simulink model "B2B_2x15kW_LCO_paralelo_y_serie"  (R2026b)
settings: Solver=ode5  StopTime=inf  EnableMultiTasking=on
StopFcn:
  | Modelo_Disable_B2B
undefined symbols (not defined in the file): ALPHA_DC, COS_RO, dataStateMachine, DiscIntNeverNeededParam, dq2abc, EN_G, getNormalizedOffset, I_MAX_G, INV_SIN_RO, KAW_CCG, KAW_DC, KI_CCG, KI_DC, KI_PLLG, KP_CCG, KP_DC, KP_PLLG, L12, LIMIT_SAG_DETECT, magnitude, MIN_VDC_READY, Ncount, NDELAY_SAG_DETECT, PORC_DC_STEADS, SAMPLES_SAG_DETECT, simDCcontCurrent1, simDCcontCurrent2, SN_G, Transformations_blocks, ts, Ts_al, TS_C, TS_PLL, UDC_min_al, UDC_Ref_al, VDC_REF, WN_G
libraries: simulink x15, TriPhaseDriveControl x13, powerlib_extras x2, model_hardware_PM15F80C_rev x2, TriphaseXenomaiTarget x1
(part 2 of 4)

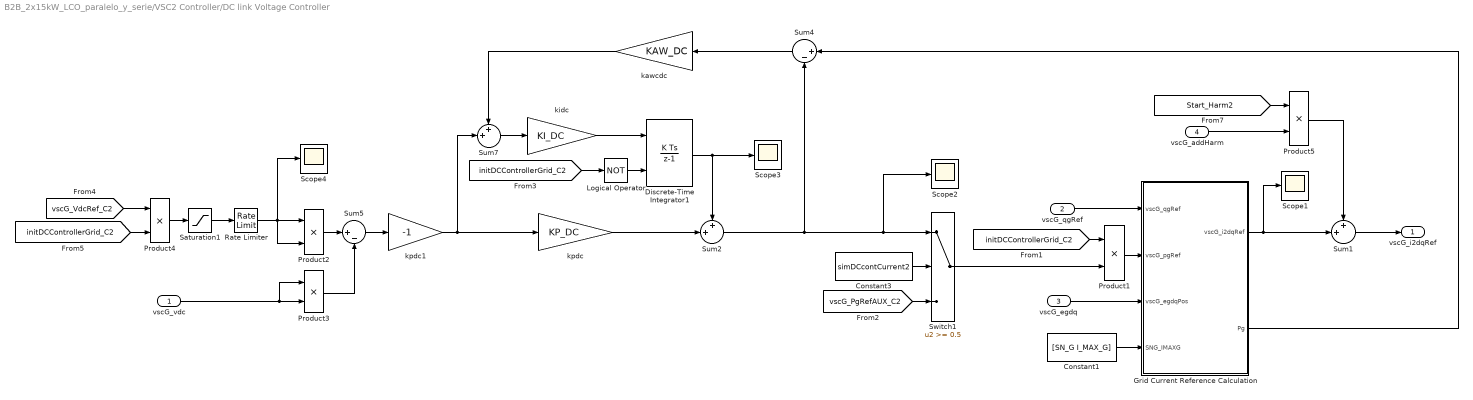
== system B2B_2x15kW_LCO_paralelo_y_serie/VSC2 Controller/DC link Voltage Controller ==
  vscG_vdc : Inport
  vscG_qgRef : Inport  Port=2
  vscG_egdq : Inport  Port=3
  vscG_addHarm : Inport  Port=4
  Constant1 : Constant  Value=[SN_G I_MAX_G]  SampleTime=TS_C
  Constant3 : Constant  Value=simDCcontCurrent2  SampleTime=TS_C
  Discrete-Time Integrator1 : DiscreteIntegrator  ExternalReset=level  SampleTime=-1  UpperSaturationLimit=sqrt(2/3)*750  LowerSaturationLimit=-sqrt(2/3)*750  ICPrevOutput=DiscIntNeverNeededParam  ICPrevScaledInput=DiscIntNeverNeededParam
  Grid Current Reference Calculation : MATLAB Function  TreatAsAtomicUnit=on
  Logical Operator : Logic  Operator=NOT  AllPortsSameDT=off  OutDataTypeStr=boolean
  Product1 : Product  RndMeth=Zero
  Product2 : Product  SaturateOnIntegerOverflow=on  OutDataTypeStr=Inherit: Same as first input
  Product3 : Product  SaturateOnIntegerOverflow=on  OutDataTypeStr=Inherit: Same as first input
  Product4 : Product  SaturateOnIntegerOverflow=on  OutDataTypeStr=Inherit: Same as first input
  Product5 : Product  RndMeth=Zero
  Rate Limiter : RateLimiter  RisingSlewLimit=500/1  FallingSlewLimit=-500/1  SampleTimeMode=inherited  InitialCondition=EN_G*sqrt(2)
  Saturation1 : Saturate  UpperLimit=VDC_REF*1.1  LowerLimit=EN_G*sqrt(2)
  Scope{1..4} (4 alike) : Scope
      Scope1 settings: SampleTime=TS_C  TimeSpan=10  ActiveDisplayYMinimum=-0  ActiveDisplayYMaximum=22  DataLoggingDecimation=5  DataLoggingVariableName=Variables_i2dq2  DataLoggingSaveFormat=Array
      Scope2 settings: SampleTime=TS_C  TimeSpan=5  ActiveDisplayYMinimum=-30000  ActiveDisplayYMaximum=2500  DataLoggingDecimation=5  DataLoggingVariableName=Variables_i2dq4  DataLoggingSaveFormat=Array
      Scope3 settings: SampleTime=TS_C  TimeSpan=5  ActiveDisplayYMinimum=24681.8  ActiveDisplayYMaximum=27279.8  DataLoggingDecimation=5  DataLoggingVariableName=Variables_i2dq5  DataLoggingSaveFormat=Array
      Scope4 settings: SampleTime=TS_C  TimeSpan=5  ActiveDisplayYMinimum=675  ActiveDisplayYMaximum=680  DataLoggingDecimation=5  DataLoggingVariableName=Variables_i2dq6  DataLoggingSaveFormat=Array
  Sum1 : Sum  Inputs=++|  InputSameDT=on  SaturateOnIntegerOverflow=on  OutDataTypeStr=Inherit: Same as first input
  Sum2 : Sum  Inputs=++|  InputSameDT=on  SaturateOnIntegerOverflow=on  OutDataTypeStr=Inherit: Same as first input
  Sum4 : Sum  Inputs=|+-  InputSameDT=on  SaturateOnIntegerOverflow=on  OutDataTypeStr=Inherit: Same as first input
  Sum5 : Sum  Inputs=|+-  InputSameDT=on  SaturateOnIntegerOverflow=on  OutDataTypeStr=Inherit: Same as first input
  Sum7 : Sum  Inputs=++|  InputSameDT=on  SaturateOnIntegerOverflow=on  OutDataTypeStr=Inherit: Same as first input
  Switch1 : Switch  Threshold=0.5  SaturateOnIntegerOverflow=off  InputSameDT=off
  kawcdc : Gain  Gain=KAW_DC  SaturateOnIntegerOverflow=on  OutDataTypeStr=Inherit: Same as input  ParamDataTypeStr=Inherit: Same as input
  kidc : Gain  Gain=KI_DC  SaturateOnIntegerOverflow=on  OutDataTypeStr=Inherit: Same as input  ParamDataTypeStr=Inherit: Same as input
  kpdc : Gain  Gain=KP_DC  SaturateOnIntegerOverflow=on  OutDataTypeStr=Inherit: Same as input  ParamDataTypeStr=Inherit: Same as input
  kpdc1 : Gain  Gain=-1  SaturateOnIntegerOverflow=on  OutDataTypeStr=Inherit: Same as input  ParamDataTypeStr=Inherit: Same as input
  vscG_i2dqRef : Outport
  wires:
  kidc/1 -> Discrete-Time Integrator1/1
  Grid Current Reference Calculation/1(vscG_i2dqRef) -> Sum1/2, Scope1/1
  vscG_egdq/1 -> Grid Current Reference Calculation/3(vscG_egdqPos)
  Constant1/1 -> Grid Current Reference Calculation/4(SNG_IMAXG)
  Logical Operator/1 -> Discrete-Time Integrator1/2
  [initDCControllerGrid_C2] -> Logical Operator/1
  [initDCControllerGrid_C2] -> Product1/1
  Product1/1 -> Grid Current Reference Calculation/2(vscG_pgRef)
  Constant3/1 -> Switch1/2
  [vscG_PgRefAUX_C2] -> Switch1/3
  Sum5/1 -> kpdc1/1
  Product3/1 -> Sum5/2
  Product2/1 -> Sum5/1
  vscG_vdc/1 -> Product3/1, Product3/2
  kpdc/1 -> Sum2/2
  Discrete-Time Integrator1/1 -> Scope3/1, Sum2/1
  Sum7/1 -> kidc/1
  Sum2/1 -> Sum4/2, Scope2/1, Switch1/1
  Sum4/1 -> kawcdc/1
  kawcdc/1 -> Sum7/1
  Grid Current Reference Calculation/2(Pg) -> Sum4/1
  vscG_qgRef/1 -> Grid Current Reference Calculation/1(vscG_qgRef)
  Switch1/1 -> Product1/2
  kpdc1/1 -> Sum7/2, kpdc/1
  Rate Limiter/1 -> Scope4/1, Product2/2, Product2/1
  [vscG_VdcRef_C2] -> Product4/1
  [initDCControllerGrid_C2] -> Product4/2
  Product4/1 -> Saturation1/1
  Saturation1/1 -> Rate Limiter/1
  vscG_addHarm/1 -> Product5/2
  Product5/1 -> Sum1/1
  [Start_Harm2] -> Product5/1
  Sum1/1 -> vscG_i2dqRef/1

== system B2B_2x15kW_LCO_paralelo_y_serie/VSC2 Controller/Grid Side Measurements ==
  vscG_i1abc : Inport
  vscG_i2abc : Inport  Port=2
  vscG_egabc : Inport  Port=3
  vscG_vdc_ : Inport  Port=4
  DSOGI QSG PLL : Subsystem
  abc to dq eg : Subsystem
  abc to dq i1 : Subsystem
  abc to dq i2 : Subsystem
  udc measurement : Subsystem
  vscG_i1dq : Outport
  vscG_i2dq : Outport  Port=2
  vscG_egdqPos : Outport  Port=3  SampleTime=TS_C
  vscG_thetaPLL : Outport  Port=4  SampleTime=TS_C
  vscG_vdc : Outport  Port=5
  vscG_egdq : Outport  Port=6
  vscG_omegaPLL : Outport  Port=7  SampleTime=TS_C
  wires:
  vscG_i1abc/1 -> abc to dq i1/1(vscG_i1abc)
  vscG_egabc/1 -> abc to dq eg/1(vscG_egabc), DSOGI QSG PLL/1(vscG_egabc)
  vscG_i2abc/1 -> abc to dq i2/1(vscG_i2abc)
  DSOGI QSG PLL/2(vscG_egdqPos) -> vscG_egdqPos/1
  vscG_vdc_/1 -> udc measurement/1(vscG_vdc_)
  udc measurement/1(vscG_vdc) -> vscG_vdc/1
  abc to dq eg/1(vscG_egdq) -> vscG_egdq/1
  DSOGI QSG PLL/3(vscG_omegaPLL) -> vscG_omegaPLL/1
  abc to dq i2/1(vscG_i2dq) -> vscG_i2dq/1
  abc to dq i1/1(vscG_i1dq) -> vscG_i1dq/1
  DSOGI QSG PLL/1(vscG_thetaPLL) -> vscG_thetaPLL/1, abc to dq eg/2(vscG_theta), abc to dq i2/2(vscG_theta), abc to dq i1/2(vscG_theta)

== system B2B_2x15kW_LCO_paralelo_y_serie/VSC2 Controller/Normalizacion ==
  vscG_ugabcActD : Inport
  vscG_vdc : Inport  Port=2
  Demux : Demux  Outputs=3
  Fcn : Fcn  Expr=2*u[1]/(u[2]+eps)
  Fcn1 : Fcn  Expr=2*u[1]/(u[2]+eps)
  Fcn2 : Fcn  Expr=2*u[1]/(u[2]+eps)
  Filter vdc : Subsystem
  Gain1 : Gain  Gain=1/2  SaturateOnIntegerOverflow=on  OutDataTypeStr=Inherit: Same as input  ParamDataTypeStr=Inherit: Same as input
  Manual Switch : ManualSwitch  CurrentSetting=0
  MinMax : MinMax  Function=max  Inputs=3  InputSameDT=on  SaturateOnIntegerOverflow=on
  MinMax2 : MinMax  Inputs=3  InputSameDT=on  SaturateOnIntegerOverflow=on
  Mux1 : Mux  Inputs=2
  Mux2 : Mux  Inputs=2
  Mux3 : Mux  Inputs=2
  Mux4 : Mux  Inputs=3
  Mux5 : Mux  Inputs=3
  Sum2 : Sum  InputSameDT=on  SaturateOnIntegerOverflow=on  OutDataTypeStr=Inherit: Same as first input
  Sum3 : Sum  Inputs=+-  InputSameDT=on  SaturateOnIntegerOverflow=on  OutDataTypeStr=Inherit: Same as first input
  Sum4 : Sum  Inputs=+-  InputSameDT=on  SaturateOnIntegerOverflow=on  OutDataTypeStr=Inherit: Same as first input
  Sum5 : Sum  Inputs=+-  InputSameDT=on  SaturateOnIntegerOverflow=on  OutDataTypeStr=Inherit: Same as first input
  vscG_dabc : Outport
  wires:
  vscG_vdc/1 -> Filter vdc/1(vscG_vdc)
  Sum3/1 -> Mux4/1  "vscG_pwmA"
  Sum4/1 -> Mux4/2  "vscG_pwmB"
  Sum5/1 -> Mux4/3  "vscG_pwmC"
  MinMax/1 -> Sum2/1
  MinMax2/1 -> Sum2/2
  Sum2/1 -> Gain1/1
  Fcn/1 -> Mux5/1, Sum3/1, MinMax2/1, MinMax/1
  Fcn2/1 -> MinMax/3, MinMax2/3, Sum5/1, Mux5/3
  Fcn1/1 -> Mux5/2, MinMax/2, MinMax2/2, Sum4/1
  Mux1/1 -> Fcn/1
  Mux2/1 -> Fcn1/1
  Mux3/1 -> Fcn2/1
  Demux/2 -> Mux2/1
  Demux/3 -> Mux3/1
  Demux/1 -> Mux1/1
  Gain1/1 -> Sum3/2, Sum4/2, Sum5/2
  Filter vdc/1(Out) -> Mux3/2, Mux1/2, Mux2/2
  vscG_ugabcActD/1 -> Demux/1
  Mux4/1 -> Manual Switch/2
  Mux5/1 -> Manual Switch/1
  Manual Switch/1 -> vscG_dabc/1

== system B2B_2x15kW_LCO_paralelo_y_serie/VSC2 Controller/State Machine ==
  Constant2 : Constant  Value=dataStateMachine  SampleTime=TS_C
  Constant6 : Constant  SampleTime=TS_C
  Constant8 : Constant  Value=0  SampleTime=TS_C
  Demux : Demux  Outputs=8
  Logic detection : Subsystem
  Mux : Mux  Inputs=6
  Scope2 : Scope
      settings: ActiveDisplayYMinimum=0  ActiveDisplayYMaximum=2100  DataLoggingVariableName=ScopeData12
  Scope3 : Scope
      settings: ActiveDisplayYMinimum=1.9  ActiveDisplayYMaximum=2.1  DataLoggingVariableName=ScopeData14
  State Machine : MATLAB Function  TreatAsAtomicUnit=on
  Unit Delay5 : UnitDelay  InitialCondition=zeros(1,Ncount)  SampleTime=TS_C
  Unit Delay7 : UnitDelay  InitialCondition=1  SampleTime=TS_C
  tag scope: CONNECT_GRID_CONTACT_C2=global, CONNECT_PRELOAD_CONTACT_C2=global, PWMOnGrid_C2=global, initCurrentControllerG_C2=global, initDCControllerGrid_C2=global, initPLLGrid_C2=global, initReactiveVoltageController_C2=global, selReactiveVoltageController_C2=global
  wires:
  State Machine/3(nowCounters) -> Unit Delay5/1, Scope2/1
  Mux/1 -> State Machine/2(inputs)
  Constant2/1 -> State Machine/1(data)
  Unit Delay5/1 -> State Machine/4(prevCounters)
  State Machine/2(nowState) -> Unit Delay7/1, Scope3/1
  Unit Delay7/1 -> State Machine/3(prevState)
  [MEAS_vscG_vdc_C2] -> Logic detection/1(vscG_vdc)
  State Machine/1(outputs) -> Demux/1
  [MEAS_vscG_egabc_C2] -> Logic detection/2(vscG_egabc)
  Demux/1 -> [PWMOnGrid_C2]
  Demux/2 -> [CONNECT_GRID_CONTACT_C2]
  Demux/3 -> [CONNECT_PRELOAD_CONTACT_C2]
  Demux/8 -> [initDCControllerGrid_C2]
  Demux/7 -> [initCurrentControllerG_C2]
  Demux/6 -> [initReactiveVoltageController_C2]
  Demux/5 -> [initPLLGrid_C2]
  Demux/4 -> [selReactiveVoltageController_C2]
  Constant6/1 -> Mux/1  "PRECHARGE"
  [INPUT_CONNECT_INT_C2] -> Mux/2  "CONNECT"
  Constant8/1 -> Mux/3
  Logic detection/1(VDC_READY) -> Mux/4
  Logic detection/2(VDC_STEATS) -> Mux/5
  Logic detection/3(FLAG_SAG) -> Mux/6

== system B2B_2x15kW_LCO_paralelo_y_serie/VSC2 Controller/dq to abc ==
  vscG_ugdqRef : Inport
  vscG_egdqPos : Inport  Port=2
  vscG_theta : Inport  Port=3
  Constant : Constant  Value=[WN_G L12 I_MAX_G]  SampleTime=TS_C
  Constant1 : Constant  Value=WN_G  SampleTime=TS_C
  Mux : Mux  Inputs=2
  Scope3 : Scope
      settings: SampleTime=TS_C  TimeSpan=5  ActiveDisplayYMinimum=24681.8  ActiveDisplayYMaximum=27279.8  DataLoggingDecimation=5  DataLoggingVariableName=Variables_i2dq7  DataLoggingSaveFormat=Array
  Sum : Sum  Inputs=|++
  dq to abc : Subsystem  AncestorBlock=Transformations_blocks/dq2abc
  th advance : Gain  Gain=TS_C*5/2
  udq Limitation : MATLAB Function  TreatAsAtomicUnit=on
  vscG_ugabcSat : Outport
  vscG_ugdqSat : Outport  Port=2
  wires:
  dq to abc/1(vscG_ugabcSat) -> vscG_ugabcSat/1
  Sum/1 -> dq to abc/2(vsc_thetaAdvanced)
  vscG_theta/1 -> Sum/1
  th advance/1 -> Sum/2
  Constant1/1 -> th advance/1
  Constant/1 -> udq Limitation/3(WNG_L12_IMAXG)
  vscG_egdqPos/1 -> udq Limitation/2(vscG_egdqPos)
  udq Limitation/1(vscG_ugdqSat) -> Mux/2, vscG_ugdqSat/1, dq to abc/1(vscG_ugdqSat)
  vscG_ugdqRef/1 -> Mux/1, udq Limitation/1(vscG_ugdqRef)
  Mux/1 -> Scope3/1

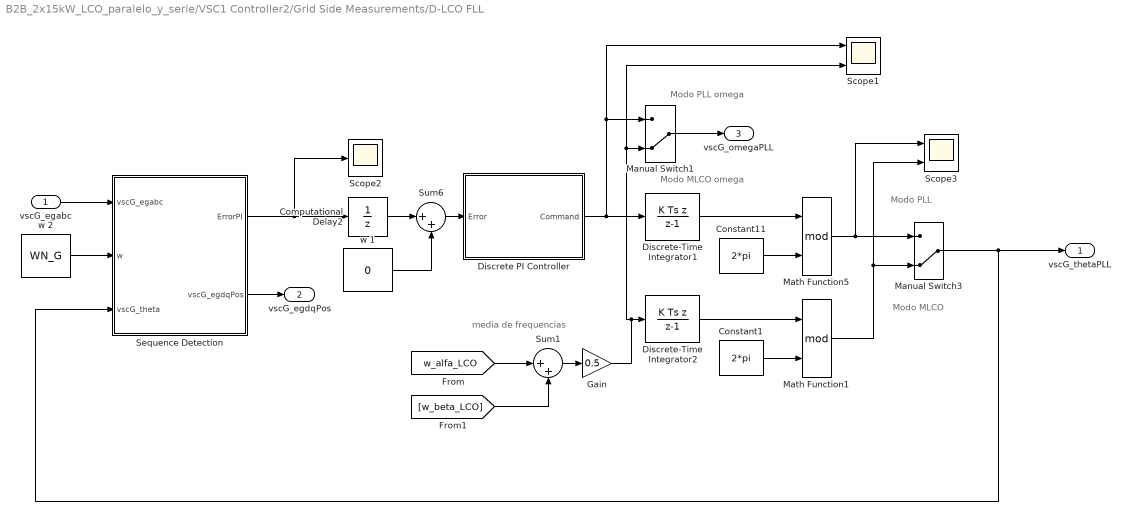
== system B2B_2x15kW_LCO_paralelo_y_serie/VSC1 Controller2/Grid Side Measurements/D-LCO FLL ==
  note: media de frequencias
  note: Modo MLCO omega
  note: Modo PLL
  note: Modo MLCO
  note: Modo PLL omega
  vscG_egabc : Inport  SampleTime=TS_PLL
  Computational Delay2 : UnitDelay  SampleTime=-1
  Constant1 : Constant  Value=2*pi  SampleTime=TS_PLL
  Constant11 : Constant  Value=2*pi  SampleTime=TS_PLL
  Discrete PI Controller : Subsystem
  Discrete-Time Integrator1 : DiscreteIntegrator  IntegratorMethod=Integration: Backward Euler  gainval=1  SampleTime=-1  ICPrevOutput=DiscIntNeverNeededParam  ICPrevScaledInput=DiscIntNeverNeededParam
  Discrete-Time Integrator2 : DiscreteIntegrator  IntegratorMethod=Integration: Backward Euler  gainval=1  SampleTime=-1  ICPrevOutput=DiscIntNeverNeededParam  ICPrevScaledInput=DiscIntNeverNeededParam
  Gain : Gain  Gain=0.5
  Manual Switch1 : ManualSwitch  CurrentSetting=0
  Manual Switch3 : ManualSwitch  CurrentSetting=0
  Math Function1 : Math  Operator=mod  SignedPower=on
  Math Function5 : Math  Operator=mod  SignedPower=on
  Scope1 : Scope  NumInputPorts=2
      settings: SampleTime=TS_C  TimeSpan=0.04  ActiveDisplayYMinimum=426200  ActiveDisplayYMaximum=426800  DataLoggingDecimation=5  DataLoggingVariableName=Variables_i2dq1  DataLoggingSaveFormat=Array
  Scope2 : Scope
      settings: SampleTime=TS_C  TimeSpan=1.978350945590096  ActiveDisplayYMinimum=-0.004  ActiveDisplayYMaximum=0.004  DataLoggingDecimation=5  DataLoggingVariableName=Variables_i2dq3  DataLoggingSaveFormat=Array
  Scope3 : Scope  NumInputPorts=2
      settings: SampleTime=TS_C  TimeSpan=0.08  ActiveDisplayYMinimum=0  ActiveDisplayYMaximum=7  DataLoggingDecimation=5  DataLoggingVariableName=Variables_i2dq  DataLoggingSaveFormat=Array
  Sequence Detection : Subsystem
  Sum1 : Sum  Inputs=|++  InputSameDT=on  SaturateOnIntegerOverflow=on  OutDataTypeStr=Inherit: Same as first input
  Sum6 : Sum  Inputs=|++  InputSameDT=on  SaturateOnIntegerOverflow=on  OutDataTypeStr=Inherit: Same as first input
  w 1 : Constant  Value=0  SampleTime=TS_PLL
  w 2 : Constant  Value=WN_G  SampleTime=TS_PLL
  vscG_thetaPLL : Outport
  vscG_egdqPos : Outport  Port=2
  vscG_omegaPLL : Outport  Port=3
  wires:
  Discrete-Time Integrator2/1 -> Math Function1/1
  Manual Switch1/1 -> vscG_omegaPLL/1
  Math Function1/1 -> Manual Switch3/2, Scope3/2
  Constant1/1 -> Math Function1/2
  Sum1/1 -> Gain/1
  Math Function5/1 -> Manual Switch3/1, Scope3/1
  Constant11/1 -> Math Function5/2
  Discrete-Time Integrator1/1 -> Math Function5/1
  Sum6/1 -> Discrete PI Controller/1(Error)
  Sequence Detection/1(ErrorPI) -> Scope2/1, Computational Delay2/1
  Discrete PI Controller/1(Command) -> Discrete-Time Integrator1/1, Manual Switch1/1, Scope1/1
  Sequence Detection/2(vscG_egdqPos) -> vscG_egdqPos/1
  Manual Switch3/1 -> vscG_thetaPLL/1, Sequence Detection/3(vscG_theta)
  Computational Delay2/1 -> Sum6/1
  vscG_egabc/1 -> Sequence Detection/1(vscG_egabc)
  w 2/1 -> Sequence Detection/2(w)
  w 1/1 -> Sum6/2
  [w_alfa_LCO] -> Sum1/1
  [w_beta_LCO] -> Sum1/2
  Gain/1 -> Manual Switch1/2, Scope1/2, Discrete-Time Integrator2/1

== system B2B_2x15kW_LCO_paralelo_y_serie/VSC1 Controller2/Grid Side Measurements/abc to dq eg ==
  vscG_egabc : Inport  SampleTime=TS_C
  vscG_theta : Inport  Port=2  SampleTime=TS_C
  Fcn3 : Fcn  Expr=u[1]*cos(u[3])+u[2]*sin(u[3])
  Fcn4 : Fcn  Expr=-u[1]*sin(u[3])+u[2]*cos(u[3])
  Fcn5 : Fcn  Expr=2/3*(u[1]-1/2*u[2]-1/2*u[3])
  Fcn6 : Fcn  Expr=2/3*(sqrt(3)/2*u[2]-sqrt(3)/2*u[3])
  Mux2 : Mux  Inputs=3
  Mux6 : Mux  Inputs=2
  vscG_egdq : Outport
  wires:
  Fcn5/1 -> Mux2/1
  Fcn6/1 -> Mux2/2
  Fcn4/1 -> Mux6/2
  Fcn3/1 -> Mux6/1
  Mux6/1 -> vscG_egdq/1
  Mux2/1 -> Fcn4/1, Fcn3/1
  vscG_egabc/1 -> Fcn6/1, Fcn5/1
  vscG_theta/1 -> Mux2/3

== system B2B_2x15kW_LCO_paralelo_y_serie/VSC1 Controller2/Grid Side Measurements/abc to dq i1 ==
  vscG_i1abc : Inport
  vscG_theta : Inport  Port=2  SampleTime=TS_C
  Fcn3 : Fcn  Expr=u[1]*cos(u[3])+u[2]*sin(u[3])
  Fcn4 : Fcn  Expr=-u[1]*sin(u[3])+u[2]*cos(u[3])
  Fcn5 : Fcn  Expr=2/3*(u[1]-1/2*u[2]-1/2*u[3])
  Fcn6 : Fcn  Expr=2/3*(sqrt(3)/2*u[2]-sqrt(3)/2*u[3])
  Mux2 : Mux  Inputs=3
  Mux6 : Mux  Inputs=2
  vscG_i1dq : Outport
  wires:
  vscG_i1abc/1 -> Fcn6/1, Fcn5/1
  Mux2/1 -> Fcn3/1, Fcn4/1
  Mux6/1 -> vscG_i1dq/1
  Fcn3/1 -> Mux6/1
  Fcn4/1 -> Mux6/2
  Fcn6/1 -> Mux2/2
  Fcn5/1 -> Mux2/1
  vscG_theta/1 -> Mux2/3

== system B2B_2x15kW_LCO_paralelo_y_serie/VSC1 Controller2/Grid Side Measurements/abc to dq i2 ==
  vscG_i2abc : Inport
  vscG_theta : Inport  Port=2  SampleTime=TS_C
  Fcn5 : Fcn  Expr=2/3*(u[1]-1/2*u[2]-1/2*u[3])
  Fcn6 : Fcn  Expr=2/3*(sqrt(3)/2*u[2]-sqrt(3)/2*u[3])
  Mux2 : Mux  Inputs=3
  Mux6 : Mux  Inputs=2
  d : Fcn  Expr=u[1]*cos(u[3])+u[2]*sin(u[3])
  q : Fcn  Expr=-u[1]*sin(u[3])+u[2]*cos(u[3])
  vscG_i2dq : Outport
  wires:
  vscG_i2abc/1 -> Fcn5/1, Fcn6/1
  Mux2/1 -> d/1, q/1
  Mux6/1 -> vscG_i2dq/1
  d/1 -> Mux6/1
  q/1 -> Mux6/2
  Fcn6/1 -> Mux2/2
  Fcn5/1 -> Mux2/1
  vscG_theta/1 -> Mux2/3

== system B2B_2x15kW_LCO_paralelo_y_serie/VSC1 Controller2/Grid Side Measurements/udc measurement ==
  note: For simulation only,
      | to avoid algebraic loop
  vscG_vdc_ : Inport
  Unit Delay1 : UnitDelay  InitialCondition=VDC_REF  SampleTime=-1
  vscG_vdc : Outport
  tag scope: MEAS_vscG_vdc_C1=global
  wires:
  Unit Delay1/1 -> [MEAS_vscG_vdc_C1], vscG_vdc/1
  vscG_vdc_/1 -> Unit Delay1/1

== system B2B_2x15kW_LCO_paralelo_y_serie/VSC1 Controller2/Normalizacion/Filter vdc ==
  vscG_vdc : Inport
  Gain2 : Gain  Gain=(1-ALPHA_DC)^2
  Gain3 : Gain  Gain=ALPHA_DC
  Gain5 : Gain  Gain=ALPHA_DC
  Sum1 : Sum
  Sum2 : Sum
  Unit Delay2 : UnitDelay  SampleTime=-1
  Unit Delay3 : UnitDelay  SampleTime=-1
  Out : Outport  PortDimensions=1
  wires:
  Gain3/1 -> Sum1/1
  Unit Delay2/1 -> Gain3/1
  Sum1/1 -> Unit Delay2/1, Sum2/2
  Gain2/1 -> Sum1/2
  vscG_vdc/1 -> Gain2/1
  Sum2/1 -> Unit Delay3/1, Out/1
  Unit Delay3/1 -> Gain5/1
  Gain5/1 -> Sum2/1

== system B2B_2x15kW_LCO_paralelo_y_serie/VSC1 Controller2/State Machine/Logic detection ==
  vscG_vdc : Inport  SampleTime=TS_C
  vscG_egabc : Inport  Port=2  SampleTime=TS_C
  Logic Conditions  VDC : Subsystem
  Sag Detection : Subsystem
  VDC_READY : Outport  SampleTime=TS_C
  VDC_STEATS : Outport  Port=2  SampleTime=TS_C
  FLAG_SAG : Outport  Port=3  SampleTime=TS_C
  wires:
  vscG_vdc/1 -> Logic Conditions  VDC/1(vscG_vdc)
  Logic Conditions  VDC/1(VDC_READY) -> VDC_READY/1
  Sag Detection/1(FLAG_SAG) -> FLAG_SAG/1
  vscG_egabc/1 -> Sag Detection/1(vscG_egabc)
  Logic Conditions  VDC/2(VDC_STEADS) -> VDC_STEATS/1

== system B2B_2x15kW_LCO_paralelo_y_serie/VSC1 Controller2/dq to abc/dq to abc ==
  vscG_ugdqSat : Inport
  vsc_thetaAdvanced : Inport  Port=2
  Mux : Mux  Inputs=2
  Mux1 : Mux  Inputs=2
  Mux2 : Mux  Inputs=3
  a : Fcn  Expr=u(1)
  alpha : Fcn  Expr=cos(u(3))*u(1)-sin(u(3))*u(2)
  b : Fcn  Expr=-0.5*u(1)+sin(2*pi/3)*u(2)
  beta : Fcn  Expr=cos(u(3))*u(2)+sin(u(3))*u(1)
  c : Fcn  Expr=-0.5*u(1)-sin(2*pi/3)*u(2)
  vscG_ugabcSat : Outport
  wires:
  Mux2/1 -> vscG_ugabcSat/1
  Mux1/1 -> c/1, b/1, a/1
  vscG_ugdqSat/1 -> Mux/1
  Mux/1 -> alpha/1, beta/1
  alpha/1 -> Mux1/1
  beta/1 -> Mux1/2
  c/1 -> Mux2/3
  b/1 -> Mux2/2
  a/1 -> Mux2/1
  vsc_thetaAdvanced/1 -> Mux/2

== system B2B_2x15kW_LCO_paralelo_y_serie/VSC2 Controller/Grid Side Measurements/DSOGI QSG PLL ==
  vscG_egabc : Inport  SampleTime=TS_PLL
  Computational Delay2 : UnitDelay  SampleTime=-1
  Constant11 : Constant  Value=2*pi  SampleTime=TS_PLL
  Discrete PI Controller : Subsystem
  Discrete-Time Integrator1 : DiscreteIntegrator  IntegratorMethod=Integration: Backward Euler  gainval=1  SampleTime=-1  ICPrevOutput=DiscIntNeverNeededParam  ICPrevScaledInput=DiscIntNeverNeededParam
  Math Function5 : Math  Operator=mod  SignedPower=on
  Scope1 : Scope
      settings: SampleTime=TS_C  TimeSpan=0.04  ActiveDisplayYMinimum=292.5  ActiveDisplayYMaximum=330  DataLoggingDecimation=5  DataLoggingVariableName=Variables_i2dq1  DataLoggingSaveFormat=Array
  Scope2 : Scope
      settings: SampleTime=TS_C  TimeSpan=1.978350945590096  ActiveDisplayYMinimum=-0.05  ActiveDisplayYMaximum=0.045  DataLoggingDecimation=5  DataLoggingVariableName=Variables_i2dq3  DataLoggingSaveFormat=Array
  Sequence Detection : Subsystem
  Sum6 : Sum  Inputs=|++  InputSameDT=on  SaturateOnIntegerOverflow=on  OutDataTypeStr=Inherit: Same as first input
  w 1 : Constant  Value=0  SampleTime=TS_PLL
  w 2 : Constant  Value=WN_G  SampleTime=TS_PLL
  vscG_thetaPLL : Outport
  vscG_egdqPos : Outport  Port=2
  vscG_omegaPLL : Outport  Port=3
  wires:
  Constant11/1 -> Math Function5/2
  Discrete-Time Integrator1/1 -> Math Function5/1
  Sum6/1 -> Discrete PI Controller/1(Error)
  Sequence Detection/1(ErrorPI) -> Scope2/1, Computational Delay2/1
  Discrete PI Controller/1(Command) -> Discrete-Time Integrator1/1, Scope1/1, vscG_omegaPLL/1
  Sequence Detection/2(vscG_egdqPos) -> vscG_egdqPos/1
  Math Function5/1 -> vscG_thetaPLL/1, Sequence Detection/3(vscG_theta)
  Computational Delay2/1 -> Sum6/1
  vscG_egabc/1 -> Sequence Detection/1(vscG_egabc)
  w 2/1 -> Sequence Detection/2(w)
  w 1/1 -> Sum6/2

== system B2B_2x15kW_LCO_paralelo_y_serie/VSC2 Controller/Grid Side Measurements/abc to dq eg ==
  vscG_egabc : Inport  SampleTime=TS_C
  vscG_theta : Inport  Port=2  SampleTime=TS_C
  Fcn3 : Fcn  Expr=u[1]*cos(u[3])+u[2]*sin(u[3])
  Fcn4 : Fcn  Expr=-u[1]*sin(u[3])+u[2]*cos(u[3])
  Fcn5 : Fcn  Expr=2/3*(u[1]-1/2*u[2]-1/2*u[3])
  Fcn6 : Fcn  Expr=2/3*(sqrt(3)/2*u[2]-sqrt(3)/2*u[3])
  Mux2 : Mux  Inputs=3
  Mux6 : Mux  Inputs=2
  vscG_egdq : Outport
  wires:
  Fcn5/1 -> Mux2/1
  Fcn6/1 -> Mux2/2
  Fcn4/1 -> Mux6/2
  Fcn3/1 -> Mux6/1
  Mux6/1 -> vscG_egdq/1
  Mux2/1 -> Fcn4/1, Fcn3/1
  vscG_egabc/1 -> Fcn6/1, Fcn5/1
  vscG_theta/1 -> Mux2/3

== system B2B_2x15kW_LCO_paralelo_y_serie/VSC2 Controller/Grid Side Measurements/abc to dq i1 ==
  vscG_i1abc : Inport
  vscG_theta : Inport  Port=2  SampleTime=TS_C
  Fcn3 : Fcn  Expr=u[1]*cos(u[3])+u[2]*sin(u[3])
  Fcn4 : Fcn  Expr=-u[1]*sin(u[3])+u[2]*cos(u[3])
  Fcn5 : Fcn  Expr=2/3*(u[1]-1/2*u[2]-1/2*u[3])
  Fcn6 : Fcn  Expr=2/3*(sqrt(3)/2*u[2]-sqrt(3)/2*u[3])
  Mux2 : Mux  Inputs=3
  Mux6 : Mux  Inputs=2
  vscG_i1dq : Outport
  wires:
  vscG_i1abc/1 -> Fcn6/1, Fcn5/1
  Mux2/1 -> Fcn3/1, Fcn4/1
  Mux6/1 -> vscG_i1dq/1
  Fcn3/1 -> Mux6/1
  Fcn4/1 -> Mux6/2
  Fcn6/1 -> Mux2/2
  Fcn5/1 -> Mux2/1
  vscG_theta/1 -> Mux2/3

== system B2B_2x15kW_LCO_paralelo_y_serie/VSC2 Controller/Grid Side Measurements/abc to dq i2 ==
  vscG_i2abc : Inport
  vscG_theta : Inport  Port=2  SampleTime=TS_C
  Fcn5 : Fcn  Expr=2/3*(u[1]-1/2*u[2]-1/2*u[3])
  Fcn6 : Fcn  Expr=2/3*(sqrt(3)/2*u[2]-sqrt(3)/2*u[3])
  Mux2 : Mux  Inputs=3
  Mux6 : Mux  Inputs=2
  d : Fcn  Expr=u[1]*cos(u[3])+u[2]*sin(u[3])
  q : Fcn  Expr=-u[1]*sin(u[3])+u[2]*cos(u[3])
  vscG_i2dq : Outport
  wires:
  vscG_i2abc/1 -> Fcn5/1, Fcn6/1
  Mux2/1 -> d/1, q/1
  Mux6/1 -> vscG_i2dq/1
  d/1 -> Mux6/1
  q/1 -> Mux6/2
  Fcn6/1 -> Mux2/2
  Fcn5/1 -> Mux2/1
  vscG_theta/1 -> Mux2/3

== system B2B_2x15kW_LCO_paralelo_y_serie/VSC2 Controller/Grid Side Measurements/udc measurement ==
  note: For simulation only,
      | to avoid algebraic loop
  vscG_vdc_ : Inport
  Unit Delay1 : UnitDelay  InitialCondition=VDC_REF  SampleTime=-1
  vscG_vdc : Outport
  tag scope: MEAS_vscG_vdc_C2=global
  wires:
  Unit Delay1/1 -> [MEAS_vscG_vdc_C2], vscG_vdc/1
  vscG_vdc_/1 -> Unit Delay1/1

== system B2B_2x15kW_LCO_paralelo_y_serie/VSC2 Controller/Normalizacion/Filter vdc ==
  vscG_vdc : Inport
  Gain2 : Gain  Gain=(1-ALPHA_DC)^2
  Gain3 : Gain  Gain=ALPHA_DC
  Gain5 : Gain  Gain=ALPHA_DC
  Sum1 : Sum
  Sum2 : Sum
  Unit Delay2 : UnitDelay  SampleTime=-1
  Unit Delay3 : UnitDelay  SampleTime=-1
  Out : Outport  PortDimensions=1
  wires:
  Gain3/1 -> Sum1/1
  Unit Delay2/1 -> Gain3/1
  Sum1/1 -> Unit Delay2/1, Sum2/2
  Gain2/1 -> Sum1/2
  vscG_vdc/1 -> Gain2/1
  Sum2/1 -> Unit Delay3/1, Out/1
  Unit Delay3/1 -> Gain5/1
  Gain5/1 -> Sum2/1

== system B2B_2x15kW_LCO_paralelo_y_serie/VSC2 Controller/State Machine/Logic detection ==
  vscG_vdc : Inport  SampleTime=TS_C
  vscG_egabc : Inport  Port=2  SampleTime=TS_C
  Logic Conditions  VDC : Subsystem
  Sag Detection : Subsystem
  VDC_READY : Outport  SampleTime=TS_C
  VDC_STEATS : Outport  Port=2  SampleTime=TS_C
  FLAG_SAG : Outport  Port=3  SampleTime=TS_C
  wires:
  vscG_vdc/1 -> Logic Conditions  VDC/1(vscG_vdc)
  Logic Conditions  VDC/1(VDC_READY) -> VDC_READY/1
  Sag Detection/1(FLAG_SAG) -> FLAG_SAG/1
  vscG_egabc/1 -> Sag Detection/1(vscG_egabc)
  Logic Conditions  VDC/2(VDC_STEADS) -> VDC_STEATS/1

== system B2B_2x15kW_LCO_paralelo_y_serie/VSC2 Controller/dq to abc/dq to abc ==
  vscG_ugdqSat : Inport
  vsc_thetaAdvanced : Inport  Port=2
  Mux : Mux  Inputs=2
  Mux1 : Mux  Inputs=2
  Mux2 : Mux  Inputs=3
  a : Fcn  Expr=u(1)
  alpha : Fcn  Expr=cos(u(3))*u(1)-sin(u(3))*u(2)
  b : Fcn  Expr=-0.5*u(1)+sin(2*pi/3)*u(2)
  beta : Fcn  Expr=cos(u(3))*u(2)+sin(u(3))*u(1)
  c : Fcn  Expr=-0.5*u(1)-sin(2*pi/3)*u(2)
  vscG_ugabcSat : Outport
  wires:
  Mux2/1 -> vscG_ugabcSat/1
  Mux1/1 -> c/1, b/1, a/1
  vscG_ugdqSat/1 -> Mux/1
  Mux/1 -> alpha/1, beta/1
  alpha/1 -> Mux1/1
  beta/1 -> Mux1/2
  c/1 -> Mux2/3
  b/1 -> Mux2/2
  a/1 -> Mux2/1
  vsc_thetaAdvanced/1 -> Mux/2

== system B2B_2x15kW_LCO_paralelo_y_serie/VSC1 Controller2/Grid Side Measurements/D-LCO FLL/Discrete PI Controller ==
  Error : Inport
  Discrete-Time Integrator : DiscreteIntegrator  ExternalReset=level  InitialCondition=49.5*2*pi  SampleTime=-1  ICPrevOutput=DiscIntNeverNeededParam  ICPrevScaledInput=DiscIntNeverNeededParam
  Kp4 : Gain  Gain=KP_PLLG  SaturateOnIntegerOverflow=on  OutDataTypeStr=Inherit: Same as input  ParamDataTypeStr=Inherit: Same as input
  Kp5 : Gain  Gain=KI_PLLG  SaturateOnIntegerOverflow=on  OutDataTypeStr=Inherit: Same as input  ParamDataTypeStr=Inherit: Same as input
  Logical Operator : Logic  Operator=NOT  AllPortsSameDT=off  OutDataTypeStr=boolean
  Sum6 : Sum  InputSameDT=on  SaturateOnIntegerOverflow=on  OutDataTypeStr=Inherit: Same as first input
  Command : Outport  InitialOutput=0
  wires:
  Kp4/1 -> Sum6/1
  Kp5/1 -> Discrete-Time Integrator/1
  Sum6/1 -> Command/1
  Discrete-Time Integrator/1 -> Sum6/2
  Logical Operator/1 -> Discrete-Time Integrator/2
  [initPLLGrid_C1] -> Logical Operator/1
  Error/1 -> Kp4/1, Kp5/1

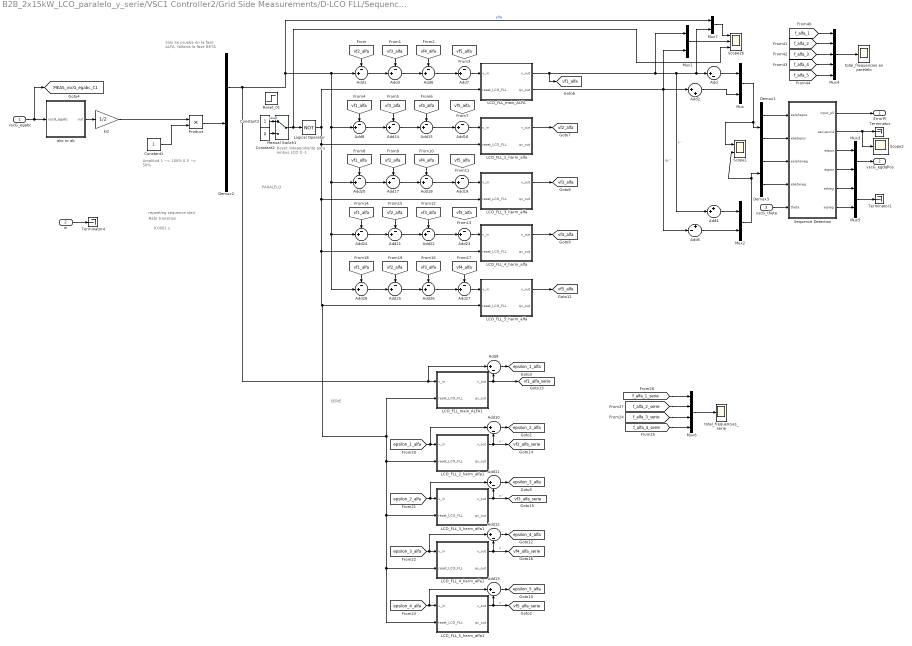
== system B2B_2x15kW_LCO_paralelo_y_serie/VSC1 Controller2/Grid Side Measurements/D-LCO FLL/Sequence Detection ==
  note: repeating sequence stair
  note: 0.0001 s
  note: Rate transition
  note: Amplitud
      | 1    --> 100%
      | 0.5 -->   50%
  note: Reset independiente
      | para ambos LCO 0 -1
  note: Sólo se prueba en la
      | fase ALFA, faltaría la fase
      | BETA
  note: PARALELO
  note: SERIE
  vscG_egabc : Inport
  w : Inport  Port=2
  vscG_theta : Inport  Port=3
  Add{,9..13} (6 alike) : Sum  Inputs=|+-
  Add{1,3,6..8,14..28} (20 alike) : Sum  Inputs=-+|
  Add2 : Sum  Inputs=|++
  Add4 : Sum  Inputs=++|
  Add5 : Sum  Inputs=+-|
  Constant1 : Constant
  Constant2 : Constant  Value=0
  Constant3 : Constant
  Demux1 : Demux  Outputs=2
  Demux2 : Demux  Outputs=2
  Demux3 : Demux  Outputs=2
  LCO_FLL_2_harm_alfa : Subsystem
  LCO_FLL_2_harm_alfa1 : Subsystem
  LCO_FLL_3_harm_alfa : Subsystem
  LCO_FLL_3_harm_alfa1 : Subsystem
  LCO_FLL_4_harm_alfa : Subsystem
  LCO_FLL_4_harm_alfa1 : Subsystem
  LCO_FLL_5_harm_alfa : Subsystem
  LCO_FLL_5_harm_alfa1 : Subsystem
  LCO_FLL_main_ALFA : Subsystem
  LCO_FLL_main_ALFA1 : Subsystem
  Logical Operator : Logic  Operator=NOT  AllPortsSameDT=off  OutDataTypeStr=boolean
  Manual Switch1 : ManualSwitch
  Mux{,1..3,5,7} (6 alike) : Mux  Inputs=2
  Mux4 : Mux  Inputs=5
  Mux6 : Mux
  Product : Product
  Reset_01 : Step  InitialValue=1  FinalValue=0  SampleTime=TS_PLL
  Scope1 : Scope  NumInputPorts=2
      settings: ActiveDisplayYMinimum=-350  ActiveDisplayYMaximum=350  DataLoggingVariableName=ScopeData3
  Scope2 : Scope
      settings: SampleTime=TS_C  TimeSpan=1.978350945590096  ActiveDisplayYMinimum=-2  ActiveDisplayYMaximum=0  DataLoggingDecimation=5  DataLoggingVariableName=Variables_i2dq8  DataLoggingSaveFormat=Array
  Scope26 : Scope  NumInputPorts=3
      settings: TimeSpan=0.1  ActiveDisplayYMinimum=-200  ActiveDisplayYMaximum=200  DataLoggingVariableName=LCO_FLL_graph
  Sequence Detection : MATLAB Function  TreatAsAtomicUnit=on
  Terminator : Terminator
  Terminator1 : Terminator
  Terminator4 : Terminator
  abc to ab : Subsystem
  ki2 : Gain  Gain=1/2
  total_frequencies en parelelo : Scope
      settings: TimeSpan=10  ActiveDisplayYMinimum=0  ActiveDisplayYMaximum=800  DataLoggingVariableName=w_LCO_paralelo
  total_frequencies_serie : Scope
      settings: TimeSpan=10  ActiveDisplayYMinimum=0  ActiveDisplayYMaximum=900  DataLoggingVariableName=w_LCO_serie_total
  ErrorPI : Outport
  vscG_egdqPos : Outport  Port=2
  tag scope: MEAS_vscG_egabc_C1=global, epsilon_1_alfa=global, epsilon_2_alfa=global, epsilon_3_alfa=global, epsilon_4_alfa=global, epsilon_5_alfa=global, vf1_alfa=global, vf1_alfa_serie=global, vf2_alfa=global, vf2_alfa_serie=global, vf3_alfa=global, vf3_alfa_serie=global, vf4_alfa=global, vf4_alfa_serie=global, vf5_alfa=global, vf5_alfa_serie=global
  wires:
  Demux3/2 -> Sequence Detection/4(ebetaneg)
  Demux3/1 -> Sequence Detection/3(ealphaneg)
  LCO_FLL_main_ALFA/1(v_out) -> [vf1_alfa], Mux1/1, Mux7/2, Add/1, Add4/2  "v '"
  LCO_FLL_main_ALFA/2(qv_out) -> Mux1/2, Add5/2, Add2/1  "qv '"
  Add/1 -> Mux/1
  Add2/1 -> Mux/2
  Add4/1 -> Mux2/1
  Add5/1 -> Mux2/2
  abc to ab/1(out) -> ki2/1
  vscG_egabc/1 -> abc to ab/1(vscG_egabc), [MEAS_vscG_egabc_C1]
  ki2/1 -> Product/1
  vscG_theta/1 -> Sequence Detection/5(theta)
  Sequence Detection/3(edpos) -> Mux3/1
  Sequence Detection/4(eqpos) -> Mux3/2
  Mux3/1 -> vscG_egdqPos/1
  Sequence Detection/5(edneg) -> Mux5/1
  Sequence Detection/6(eqneg) -> Mux5/2
  Mux/1 -> Demux1/1, Scope1/1
  Mux2/1 -> Scope1/2, Demux3/1
  Sequence Detection/2(secuencia) -> Terminator/1, Scope2/1
  Mux5/1 -> Terminator1/1
  Demux1/1 -> Sequence Detection/1(ealphapos)
  Demux1/2 -> Sequence Detection/2(ebetapos)
  Sequence Detection/1(input_pll) -> ErrorPI/1
  Mux1/1 -> Scope26/2
  w/1 -> Terminator4/1
  Mux7/1 -> Scope26/1
  Manual Switch1/1 -> Scope26/3, Logical Operator/1
  Constant1/1 -> Product/2
  Product/1 -> Demux2/1
  Constant3/1 -> Manual Switch1/1  "reset"
  Constant2/1 -> Manual Switch1/2
  LCO_FLL_2_harm_alfa/1(v_out) -> [vf2_alfa]
  LCO_FLL_3_harm_alfa/1(v_out) -> [vf3_alfa]
  LCO_FLL_4_harm_alfa/1(v_out) -> [vf4_alfa]
  LCO_FLL_5_harm_alfa/1(v_out) -> [vf5_alfa]
  Add1/1 -> Add3/2
  Add3/1 -> Add6/2
  Add6/1 -> Add7/2
  Add7/1 -> LCO_FLL_main_ALFA/1(v_in)
  [vf2_alfa] -> Add1/1
  [vf3_alfa] -> Add3/1
  [vf4_alfa] -> Add6/1
  Add8/1 -> Add14/2
  Add14/1 -> Add15/2
  Add15/1 -> Add16/2
  [vf1_alfa] -> Add8/1
  [vf3_alfa] -> Add14/1
  [vf4_alfa] -> Add15/1
  Add16/1 -> LCO_FLL_2_harm_alfa/1(v_in)
  Add20/1 -> Add17/2
  Add17/1 -> Add18/2
  Add18/1 -> Add19/2
  [vf1_alfa] -> Add20/1
  [vf2_alfa] -> Add17/1
  [vf4_alfa] -> Add18/1
  Add19/1 -> LCO_FLL_3_harm_alfa/1(v_in)
  Add24/1 -> Add21/2
  Add21/1 -> Add22/2
  Add22/1 -> Add23/2
  [vf1_alfa] -> Add24/1
  [vf2_alfa] -> Add21/1
  [vf3_alfa] -> Add22/1
  Add23/1 -> LCO_FLL_4_harm_alfa/1(v_in)
  Add28/1 -> Add25/2
  Add25/1 -> Add26/2
  Add26/1 -> Add27/2
  [vf1_alfa] -> Add28/1
  [vf2_alfa] -> Add25/1
  [vf3_alfa] -> Add26/1
  [vf4_alfa] -> Add27/1
  Add27/1 -> LCO_FLL_5_harm_alfa/1(v_in)
  Mux4/1 -> total_frequencies en parelelo/1
  [f_alfa_1] -> Mux4/1
  [f_alfa_2] -> Mux4/2
  [f_alfa_3] -> Mux4/3
  [f_alfa_4] -> Mux4/4
  [f_alfa_5] -> Mux4/5
  LCO_FLL_main_ALFA1/1(v_out) -> [vf1_alfa_serie], Add9/2
  Demux2/1 -> Add9/1, LCO_FLL_main_ALFA1/1(v_in), Add28/2, Add24/2, Add20/2, Add8/2, Add1/2, Mux7/1  "alfa"
  Add9/1 -> [epsilon_1_alfa]
  [epsilon_1_alfa] -> Add10/1, LCO_FLL_2_harm_alfa1/1(v_in)
  LCO_FLL_2_harm_alfa1/1(v_out) -> [vf2_alfa_serie], Add10/2  "v '"
  Add10/1 -> [epsilon_2_alfa]
  [epsilon_2_alfa] -> Add11/1, LCO_FLL_3_harm_alfa1/1(v_in)
  [epsilon_3_alfa] -> Add12/1, LCO_FLL_4_harm_alfa1/1(v_in)
  LCO_FLL_3_harm_alfa1/1(v_out) -> [vf3_alfa_serie], Add11/2  "v '"
  Add11/1 -> [epsilon_3_alfa]
  LCO_FLL_4_harm_alfa1/1(v_out) -> [vf4_alfa_serie], Add12/2  "v '"
  Add12/1 -> [epsilon_4_alfa]
  [epsilon_4_alfa] -> LCO_FLL_5_harm_alfa1/1(v_in), Add13/1
  LCO_FLL_5_harm_alfa1/1(v_out) -> [vf5_alfa_serie], Add13/2  "v '"
  Add13/1 -> [epsilon_5_alfa]
  Logical Operator/1 -> LCO_FLL_2_harm_alfa/2(reset_LCO_FLL), LCO_FLL_3_harm_alfa/2(reset_LCO_FLL), LCO_FLL_4_harm_alfa/2(reset_LCO_FLL), LCO_FLL_2_harm_alfa1/2(reset_LCO_FLL), LCO_FLL_3_harm_alfa1/2(reset_LCO_FLL), LCO_FLL_4_harm_alfa1/2(reset_LCO_FLL), LCO_FLL_5_harm_alfa1/2(reset_LCO_FLL), LCO_FLL_main_ALFA1/2(reset_LCO_FLL), LCO_FLL_5_harm_alfa/2(reset_LCO_FLL), LCO_FLL_main_ALFA/2(reset_LCO_FLL)
  Mux6/1 -> total_frequencies_serie/1
  [f_alfa_1_serie] -> Mux6/1
  [f_alfa_2_serie] -> Mux6/2
  [f_alfa_3_serie] -> Mux6/3
  [f_alfa_4_serie] -> Mux6/4

== system B2B_2x15kW_LCO_paralelo_y_serie/VSC1 Controller2/State Machine/Logic detection/Logic Conditions  VDC ==
  vscG_vdc : Inport
  Compare To Constant1 : simulink/Logic and Bit Operations/Compare To Constant  relop=>=  const=VDC_REF*(1-PORC_DC_STEADS)  OutDataTypeStr=uint8
  Compare To Constant2 : simulink/Logic and Bit Operations/Compare To Constant  relop=<=  const=VDC_REF*(1+PORC_DC_STEADS)  OutDataTypeStr=uint8
  Compare To Constant3 : simulink/Logic and Bit Operations/Compare To Constant  relop=>=  const=MIN_VDC_READY  OutDataTypeStr=uint8
  Data Type Conversion : DataTypeConversion  SaturateOnIntegerOverflow=off  RndMeth=Floor
  Data Type Conversion1 : DataTypeConversion  SaturateOnIntegerOverflow=off  RndMeth=Floor
  Logical Operator3 : Logic  Operator=OR  AllPortsSameDT=off  OutDataTypeStr=boolean
  Unit Delay1 : UnitDelay  SampleTime=TS_C
  Unit Delay6 : UnitDelay  SampleTime=TS_C
  VDC_READY : Outport
  VDC_STEADS : Outport  Port=2
  wires:
  Data Type Conversion/1 -> Unit Delay6/1
  Compare To Constant3/1 -> Data Type Conversion/1
  vscG_vdc/1 -> Compare To Constant3/1, Compare To Constant1/1, Compare To Constant2/1
  Unit Delay6/1 -> VDC_READY/1
  Compare To Constant1/1 -> Logical Operator3/1
  Unit Delay1/1 -> Data Type Conversion1/1
  Compare To Constant2/1 -> Logical Operator3/2
  Logical Operator3/1 -> Unit Delay1/1
  Data Type Conversion1/1 -> VDC_STEADS/1

== system B2B_2x15kW_LCO_paralelo_y_serie/VSC1 Controller2/State Machine/Logic detection/Sag Detection ==
  vscG_egabc : Inport
  Constant : Constant  Value=(sqrt(2)*(EN_G/sqrt(3))*LIMIT_SAG_DETECT)^2
  Data Type Conversion : DataTypeConversion  SaturateOnIntegerOverflow=off  RndMeth=Floor
  Demux : Demux  Outputs=3
  Gain : Gain  Gain=INV_SIN_RO
  Gain1 : Gain  Gain=COS_RO
  Integer Delay : Delay  DelayLength=SAMPLES_SAG_DETECT
  Limite superior : RelationalOperator  Operator=<  OutDataTypeStr=fixdt(0,8)  InputSameDT=off
  Logical Operator : Logic  Inputs=1  AllPortsSameDT=off  OutDataTypeStr=boolean
  Logical Operator1 : Logic  Inputs=1  AllPortsSameDT=off  OutDataTypeStr=boolean
  Logical Operator2 : Logic  Inputs=1  AllPortsSameDT=off  OutDataTypeStr=boolean
  Logical Operator3 : Logic  Operator=OR  Inputs=3  AllPortsSameDT=off  OutDataTypeStr=boolean
  Math Function : Math  Operator=magnitude^2  SignedPower=on
  Math Function1 : Math  Operator=magnitude^2  SignedPower=on
  Sum : Sum  Inputs=|+-
  Sum1 : Sum
  Tapped Delay : simulink/Discrete/Tapped Delay  vinit=[zeros(NDELAY_SAG_DETECT,1)]'  samptime=-1  NumDelays=NDELAY_SAG_DETECT  DelayOrder=Oldest  includeCurrent=on
  Tapped Delay1 : simulink/Discrete/Tapped Delay  vinit=[zeros(NDELAY_SAG_DETECT,1)]'  samptime=-1  NumDelays=NDELAY_SAG_DETECT  DelayOrder=Oldest  includeCurrent=on
  Tapped Delay2 : simulink/Discrete/Tapped Delay  vinit=[zeros(NDELAY_SAG_DETECT,1)]'  samptime=-1  NumDelays=NDELAY_SAG_DETECT  DelayOrder=Oldest  includeCurrent=on
  Unit Delay2 : UnitDelay  SampleTime=-1
  FLAG_SAG : Outport
  wires:
  Gain/1 -> Gain1/1, Integer Delay/1
  Integer Delay/1 -> Sum/1
  Gain1/1 -> Sum/2
  Sum/1 -> Math Function1/1
  Math Function/1 -> Sum1/1
  Math Function1/1 -> Sum1/2
  Sum1/1 -> Limite superior/1  "vscG_egabcModPow2"
  vscG_egabc/1 -> Math Function/1, Gain/1
  Tapped Delay/1 -> Logical Operator/1
  Constant/1 -> Limite superior/2
  Limite superior/1 -> Demux/1
  Demux/1 -> Tapped Delay/1
  Tapped Delay1/1 -> Logical Operator1/1
  Demux/2 -> Tapped Delay1/1
  Tapped Delay2/1 -> Logical Operator2/1
  Logical Operator1/1 -> Logical Operator3/2
  Logical Operator/1 -> Logical Operator3/1
  Logical Operator2/1 -> Logical Operator3/3
  Demux/3 -> Tapped Delay2/1
  Logical Operator3/1 -> Data Type Conversion/1
  Data Type Conversion/1 -> Unit Delay2/1
  Unit Delay2/1 -> FLAG_SAG/1

== system B2B_2x15kW_LCO_paralelo_y_serie/VSC2 Controller/Grid Side Measurements/DSOGI QSG PLL/Discrete PI Controller ==
  Error : Inport
  Discrete-Time Integrator : DiscreteIntegrator  ExternalReset=level  InitialCondition=49.5*2*pi  SampleTime=-1  ICPrevOutput=DiscIntNeverNeededParam  ICPrevScaledInput=DiscIntNeverNeededParam
  Kp4 : Gain  Gain=KP_PLLG  SaturateOnIntegerOverflow=on  OutDataTypeStr=Inherit: Same as input  ParamDataTypeStr=Inherit: Same as input
  Kp5 : Gain  Gain=KI_PLLG  SaturateOnIntegerOverflow=on  OutDataTypeStr=Inherit: Same as input  ParamDataTypeStr=Inherit: Same as input
  Logical Operator : Logic  Operator=NOT  AllPortsSameDT=off  OutDataTypeStr=boolean
  Sum6 : Sum  InputSameDT=on  SaturateOnIntegerOverflow=on  OutDataTypeStr=Inherit: Same as first input
  Command : Outport  InitialOutput=0
  wires:
  Kp4/1 -> Sum6/1
  Kp5/1 -> Discrete-Time Integrator/1
  Sum6/1 -> Command/1
  Discrete-Time Integrator/1 -> Sum6/2
  Logical Operator/1 -> Discrete-Time Integrator/2
  [initPLLGrid_C2] -> Logical Operator/1
  Error/1 -> Kp4/1, Kp5/1

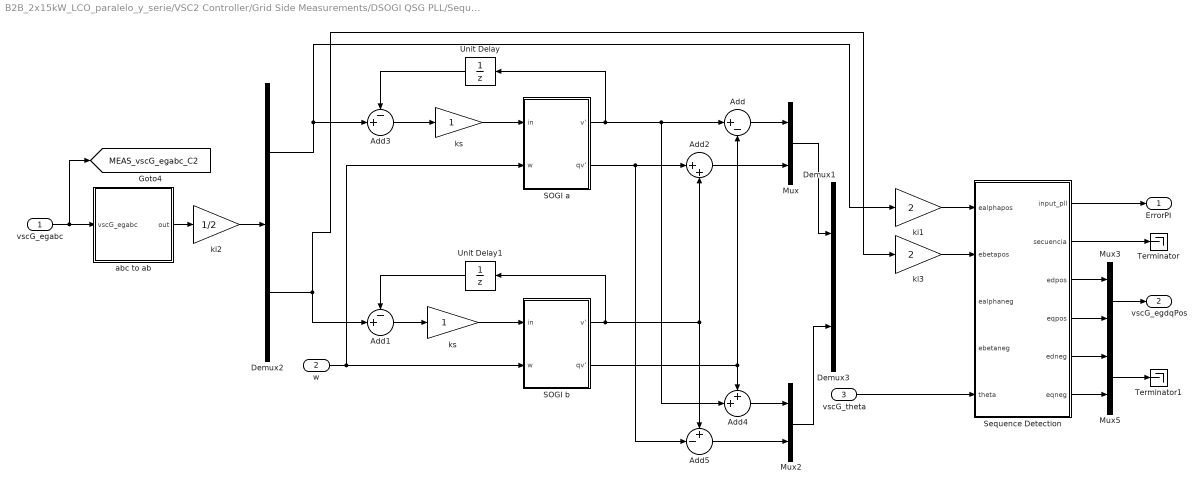
== system B2B_2x15kW_LCO_paralelo_y_serie/VSC2 Controller/Grid Side Measurements/DSOGI QSG PLL/Sequence Detection ==
  vscG_egabc : Inport
  w : Inport  Port=2
  vscG_theta : Inport  Port=3
  Add : Sum  Inputs=|+-
  Add1 : Sum  Inputs=-+|
  Add2 : Sum  Inputs=|++
  Add3 : Sum  Inputs=-+|
  Add4 : Sum  Inputs=++|
  Add5 : Sum  Inputs=+-|
  Demux1 : Demux  Outputs=2
  Demux2 : Demux  Outputs=2
  Demux3 : Demux  Outputs=2
  Mux{,2..3,5} (4 alike) : Mux  Inputs=2
  "SOGI a " : Subsystem
  SOGI b : Subsystem
  Sequence Detection : MATLAB Function  TreatAsAtomicUnit=on
  Terminator : Terminator
  Terminator1 : Terminator
  Unit Delay : UnitDelay  SampleTime=-1
  Unit Delay1 : UnitDelay  SampleTime=-1
  abc to ab : Subsystem
  ki1 : Gain  Gain=2
  ki2 : Gain  Gain=1/2
  ki3 : Gain  Gain=2
  ks : Gain
  "ks " : Gain
  ErrorPI : Outport
  vscG_egdqPos : Outport  Port=2
  tag scope: MEAS_vscG_egabc_C2=global
  wires:
  ks/1 -> "SOGI a "/1(in)
  Add3/1 -> ks/1
  "SOGI a "/1(v') -> Add/1, Add4/2, Unit Delay/1
  Unit Delay/1 -> Add3/1
  "SOGI a "/2(qv') -> Add2/1, Add5/2
  "ks "/1 -> SOGI b/1(in)
  Add1/1 -> "ks "/1
  SOGI b/1(v') -> Add5/1, Add2/2, Unit Delay1/1
  SOGI b/2(qv') -> Add4/1, Add/2
  Add/1 -> Mux/1
  Add2/1 -> Mux/2
  Add4/1 -> Mux2/1
  Add5/1 -> Mux2/2
  abc to ab/1(out) -> ki2/1
  Demux2/1 -> ki1/1, Add3/2
  Demux2/2 -> ki3/1, Add1/2
  Unit Delay1/1 -> Add1/1
  vscG_egabc/1 -> abc to ab/1(vscG_egabc), [MEAS_vscG_egabc_C2]
  ki2/1 -> Demux2/1
  vscG_theta/1 -> Sequence Detection/5(theta)
  Sequence Detection/3(edpos) -> Mux3/1
  Sequence Detection/4(eqpos) -> Mux3/2
  Mux3/1 -> vscG_egdqPos/1
  Sequence Detection/5(edneg) -> Mux5/1
  Sequence Detection/6(eqneg) -> Mux5/2
  Mux/1 -> Demux1/1
  Mux2/1 -> Demux3/1
  w/1 -> "SOGI a "/2(w), SOGI b/2(w)
  Sequence Detection/2(secuencia) -> Terminator/1
  Mux5/1 -> Terminator1/1
  Sequence Detection/1(input_pll) -> ErrorPI/1
  ki1/1 -> Sequence Detection/1(ealphapos)
  ki3/1 -> Sequence Detection/2(ebetapos)

== system B2B_2x15kW_LCO_paralelo_y_serie/VSC2 Controller/State Machine/Logic detection/Logic Conditions  VDC ==
  vscG_vdc : Inport
  Compare To Constant1 : simulink/Logic and Bit Operations/Compare To Constant  relop=>=  const=VDC_REF*(1-PORC_DC_STEADS)  OutDataTypeStr=uint8
  Compare To Constant2 : simulink/Logic and Bit Operations/Compare To Constant  relop=<=  const=VDC_REF*(1+PORC_DC_STEADS)  OutDataTypeStr=uint8
  Compare To Constant3 : simulink/Logic and Bit Operations/Compare To Constant  relop=>=  const=MIN_VDC_READY  OutDataTypeStr=uint8
  Data Type Conversion : DataTypeConversion  SaturateOnIntegerOverflow=off  RndMeth=Floor
  Data Type Conversion1 : DataTypeConversion  SaturateOnIntegerOverflow=off  RndMeth=Floor
  Logical Operator3 : Logic  Operator=OR  AllPortsSameDT=off  OutDataTypeStr=boolean
  Unit Delay1 : UnitDelay  SampleTime=TS_C
  Unit Delay6 : UnitDelay  SampleTime=TS_C
  VDC_READY : Outport
  VDC_STEADS : Outport  Port=2
  wires:
  Data Type Conversion/1 -> Unit Delay6/1
  Compare To Constant3/1 -> Data Type Conversion/1
  vscG_vdc/1 -> Compare To Constant3/1, Compare To Constant1/1, Compare To Constant2/1
  Unit Delay6/1 -> VDC_READY/1
  Compare To Constant1/1 -> Logical Operator3/1
  Unit Delay1/1 -> Data Type Conversion1/1
  Compare To Constant2/1 -> Logical Operator3/2
  Logical Operator3/1 -> Unit Delay1/1
  Data Type Conversion1/1 -> VDC_STEADS/1

== system B2B_2x15kW_LCO_paralelo_y_serie/VSC2 Controller/State Machine/Logic detection/Sag Detection ==
  vscG_egabc : Inport
  Constant : Constant  Value=(sqrt(2)*(EN_G/sqrt(3))*LIMIT_SAG_DETECT)^2
  Data Type Conversion : DataTypeConversion  SaturateOnIntegerOverflow=off  RndMeth=Floor
  Demux : Demux  Outputs=3
  Gain : Gain  Gain=INV_SIN_RO
  Gain1 : Gain  Gain=COS_RO
  Integer Delay : Delay  DelayLength=SAMPLES_SAG_DETECT
  Limite superior : RelationalOperator  Operator=<  OutDataTypeStr=fixdt(0,8)  InputSameDT=off
  Logical Operator : Logic  Inputs=1  AllPortsSameDT=off  OutDataTypeStr=boolean
  Logical Operator1 : Logic  Inputs=1  AllPortsSameDT=off  OutDataTypeStr=boolean
  Logical Operator2 : Logic  Inputs=1  AllPortsSameDT=off  OutDataTypeStr=boolean
  Logical Operator3 : Logic  Operator=OR  Inputs=3  AllPortsSameDT=off  OutDataTypeStr=boolean
  Math Function : Math  Operator=magnitude^2  SignedPower=on
  Math Function1 : Math  Operator=magnitude^2  SignedPower=on
  Sum : Sum  Inputs=|+-
  Sum1 : Sum
  Tapped Delay : simulink/Discrete/Tapped Delay  vinit=[zeros(NDELAY_SAG_DETECT,1)]'  samptime=-1  NumDelays=NDELAY_SAG_DETECT  DelayOrder=Oldest  includeCurrent=on
  Tapped Delay1 : simulink/Discrete/Tapped Delay  vinit=[zeros(NDELAY_SAG_DETECT,1)]'  samptime=-1  NumDelays=NDELAY_SAG_DETECT  DelayOrder=Oldest  includeCurrent=on
  Tapped Delay2 : simulink/Discrete/Tapped Delay  vinit=[zeros(NDELAY_SAG_DETECT,1)]'  samptime=-1  NumDelays=NDELAY_SAG_DETECT  DelayOrder=Oldest  includeCurrent=on
  Unit Delay2 : UnitDelay  SampleTime=-1
  FLAG_SAG : Outport
  wires:
  Gain/1 -> Gain1/1, Integer Delay/1
  Integer Delay/1 -> Sum/1
  Gain1/1 -> Sum/2
  Sum/1 -> Math Function1/1
  Math Function/1 -> Sum1/1
  Math Function1/1 -> Sum1/2
  Sum1/1 -> Limite superior/1  "vscG_egabcModPow2"
  vscG_egabc/1 -> Math Function/1, Gain/1
  Tapped Delay/1 -> Logical Operator/1
  Constant/1 -> Limite superior/2
  Limite superior/1 -> Demux/1
  Demux/1 -> Tapped Delay/1
  Tapped Delay1/1 -> Logical Operator1/1
  Demux/2 -> Tapped Delay1/1
  Tapped Delay2/1 -> Logical Operator2/1
  Logical Operator1/1 -> Logical Operator3/2
  Logical Operator/1 -> Logical Operator3/1
  Logical Operator2/1 -> Logical Operator3/3
  Demux/3 -> Tapped Delay2/1
  Logical Operator3/1 -> Data Type Conversion/1
  Data Type Conversion/1 -> Unit Delay2/1
  Unit Delay2/1 -> FLAG_SAG/1

== system B2B_2x15kW_LCO_paralelo_y_serie/VSC1 Controller2/Grid Side Measurements/D-LCO FLL/Sequence Detection/LCO_FLL_2_harm_alfa ==
  note: Para que no se valla a inf
  note: los regresamos
      | a la ganancia
      | original
  note: 1 sobre la ganancia
      | del interarmónico
      | 1/0.05 = 20
  v_in : Inport
  reset_LCO_FLL : Inport  Port=2
  Constant1 : Constant  Value=50
  Demux1 : Demux  Outputs=5
  Demux4 : Demux  Outputs=3
  Discrete-Time Integrator1 : DiscreteIntegrator  gainval=[1 1 1]  ExternalReset=either  InitialCondition=[1 1 10]  SampleTime=TS_PLL  ICPrevOutput=DiscIntNeverNeededParam  ICPrevScaledInput=DiscIntNeverNeededParam
  K gain : Constant  Value=0.1
  LCO_FLL_01 : MATLAB Function  TreatAsAtomicUnit=on
  Mux1 : Mux  Inputs=3
  Mux4 : Mux  Inputs=2
  Mux6 : Mux  Inputs=3
  Saturation2 : Saturate  UpperLimit=5000  LowerLimit=-5000
  Sinch 2 harm paralel : Scope
      settings: TimeSpan=0.1  ActiveDisplayYMinimum=-100  ActiveDisplayYMaximum=100  DataLoggingVariableName=LCO_FLL_graph2_paralelo
  Terminator3 : Terminator
  delta w : Scope
      settings: TimeSpan=20  ActiveDisplayYMinimum=-31  ActiveDisplayYMaximum=-24  DataLoggingVariableName=ScopeData4
  freq : Scope
      settings: TimeSpan=10  ActiveDisplayYMinimum=308  ActiveDisplayYMaximum=322  DataLoggingVariableName=w_LCO1_paralelo
  ki1 : Gain  Gain=1.8
  ki2 : Gain  Gain=1/(2*pi)
  ki3 : Gain  Gain=1/1.8
  ki4 : Gain  Gain=1/1.8
  v_out : Outport
  qv_out : Outport  Port=2
  tag scope: f_alfa_2=global
  wires:
  LCO_FLL_01/4(w) -> ki2/1
  LCO_FLL_01/3(x3p) -> Mux1/3
  LCO_FLL_01/2(x2p) -> Mux1/2
  LCO_FLL_01/1(x1p) -> Mux1/1
  Demux1/5 -> LCO_FLL_01/5(v)
  Demux1/4 -> LCO_FLL_01/4(A)
  Demux1/3 -> LCO_FLL_01/3(x3)
  Demux1/2 -> LCO_FLL_01/2(x2)
  Mux6/1 -> Demux1/1
  Demux1/1 -> LCO_FLL_01/1(x1)
  Demux4/2 -> Mux4/2, ki4/1  "x2 - v '"
  Demux4/1 -> ki3/1  "x1 - qv '"
  Demux4/3 -> Terminator3/1, delta w/1  "x3 -  delta w"
  reset_LCO_FLL/1 -> Discrete-Time Integrator1/2
  Mux1/1 -> Discrete-Time Integrator1/1
  Constant1/1 -> Mux6/2  "A"
  v_in/1 -> ki1/1
  Saturation2/1 -> Mux6/1
  Discrete-Time Integrator1/1 -> Demux4/1, Saturation2/1
  ki2/1 -> [f_alfa_2], freq/1
  Mux4/1 -> Sinch 2 harm paralel/1
  ki4/1 -> v_out/1
  ki3/1 -> qv_out/1
  ki1/1 -> Mux4/1, Mux6/3
  K gain/1 -> LCO_FLL_01/6(k)

== system B2B_2x15kW_LCO_paralelo_y_serie/VSC1 Controller2/Grid Side Measurements/D-LCO FLL/Sequence Detection/LCO_FLL_2_harm_alfa1 ==
  note: los regresamos
      | a la ganancia
      | original
  note: 1 sobre la ganancia
      | del interarmónico
      | 1/0.05 = 20
  note: Para que no se valla a inf
  v_in : Inport
  reset_LCO_FLL : Inport  Port=2
  Constant1 : Constant  Value=50
  Demux1 : Demux  Outputs=5
  Demux4 : Demux  Outputs=3
  Discrete-Time Integrator1 : DiscreteIntegrator  gainval=[1 1 1]  ExternalReset=either  InitialCondition=[1 1 10]  SampleTime=TS_PLL  ICPrevOutput=DiscIntNeverNeededParam  ICPrevScaledInput=DiscIntNeverNeededParam
  K gain : Constant  Value=0.1
  LCO_FLL_01 : MATLAB Function  TreatAsAtomicUnit=on
  Mux1 : Mux  Inputs=3
  Mux4 : Mux  Inputs=2
  Mux6 : Mux  Inputs=3
  Saturation2 : Saturate  UpperLimit=5000  LowerLimit=-5000
  Sinch 2 harm serie : Scope
      settings: TimeSpan=0.1  ActiveDisplayYMinimum=-100  ActiveDisplayYMaximum=100  DataLoggingVariableName=LCO_FLL_graph02_serie
  Terminator3 : Terminator
  delta w : Scope
      settings: TimeSpan=20  ActiveDisplayYMinimum=761.5  ActiveDisplayYMaximum=764.5  DataLoggingVariableName=ScopeData4
  freq alfa 2 : Scope
      settings: TimeSpan=10  ActiveDisplayYMinimum=0  ActiveDisplayYMaximum=1  DataLoggingVariableName=w_LCO1_serie
  ki1 : Gain  Gain=1.8
  ki2 : Gain  Gain=1/(2*pi)
  ki3 : Gain  Gain=1/1.8
  ki4 : Gain  Gain=1/1.8
  v_out : Outport
  qv_out : Outport  Port=2
  tag scope: f_alfa_2_serie=global
  wires:
  LCO_FLL_01/4(w) -> ki2/1
  LCO_FLL_01/3(x3p) -> Mux1/3
  LCO_FLL_01/2(x2p) -> Mux1/2
  LCO_FLL_01/1(x1p) -> Mux1/1
  Demux1/5 -> LCO_FLL_01/5(v)
  Demux1/4 -> LCO_FLL_01/4(A)
  Demux1/3 -> LCO_FLL_01/3(x3)
  Demux1/2 -> LCO_FLL_01/2(x2)
  Mux6/1 -> Demux1/1
  Demux1/1 -> LCO_FLL_01/1(x1)
  Demux4/2 -> Mux4/2, ki4/1  "x2 - v '"
  Demux4/1 -> ki3/1  "x1 - qv '"
  Demux4/3 -> Terminator3/1, delta w/1  "x3 -  delta w"
  reset_LCO_FLL/1 -> Discrete-Time Integrator1/2
  Mux1/1 -> Discrete-Time Integrator1/1
  Constant1/1 -> Mux6/2  "A"
  ki1/1 -> Mux4/1, Mux6/3
  Saturation2/1 -> Mux6/1
  Discrete-Time Integrator1/1 -> Demux4/1, Saturation2/1
  ki2/1 -> [f_alfa_2_serie], freq alfa 2/1
  v_in/1 -> ki1/1
  ki3/1 -> qv_out/1
  ki4/1 -> v_out/1
  Mux4/1 -> Sinch 2 harm serie/1
  K gain/1 -> LCO_FLL_01/6(k)
